simulink model "ThdRwRtStBkReclnTrgtPosSelc"  (R2018b)
settings: Solver=FixedStepDiscrete  StartTime=0.0  StopTime=10.0  RelTol=1e-3
undefined symbols (not defined in the file or in its folder): KeSMSw6sAcsEntryThdRwRtStBkReclnUpwdDnwdPos_Val, KeSMSw6sAcsEntryThdRwRtStBkReclnUpwdDnwdPosMax_Val, KeSMSw6sAcsEntryThdRwRtStBkReclnUpwdDnwdPosMin_Val, KeSMSw6sLugThdRwRtStBkReclnUpwdDnwdPos_Val, KeSMSw6sLugThdRwRtStBkReclnUpwdDnwdPosMax_Val, KeSMSw6sLugThdRwRtStBkReclnUpwdDnwdPosMin_Val, KeSMSw6sVIPThdRwRtStBkReclnUpwdDnwdPos_Val, KeSMSw6sVIPThdRwRtStBkReclnUpwdDnwdPosMax_Val, KeSMSw6sVIPThdRwRtStBkReclnUpwdDnwdPosMin_Val, KeSMSwAcsEntryThdRwRtStBkReclnUpwdDnwdPos_Val, KeSMSwAcsEntryThdRwRtStBkReclnUpwdDnwdPosMax_Val, KeSMSwAcsEntryThdRwRtStBkReclnUpwdDnwdPosMin_Val, KeSMSwAcsMd53ThdRwRtBkReclnUpwdDnwdPos_Val, KeSMSwAcsMd53ThdRwRtBkReclnUpwdDnwdPosMax_Val, KeSMSwAcsMd53ThdRwRtBkReclnUpwdDnwdPosMin_Val, KeSMSwLugThdRwRtStBkReclnUpwdDnwdPos_Val, KeSMSwLugThdRwRtStBkReclnUpwdDnwdPosMax_Val, KeSMSwLugThdRwRtStBkReclnUpwdDnwdPosMin_Val, KeSMSwVIPThdRwRtStBkReclnUpwdDnwdPos_Val, KeSMSwVIPThdRwRtStBkReclnUpwdDnwdPosMax_Val, KeSMSwVIPThdRwRtStBkReclnUpwdDnwdPosMin_Val
libraries: TrgtPosSelcLib x5
settings Model: Creator=sn2xws  LastModifiedBy=sn2xws
settings Model: ModifiedHistory=|
  | 2024.6.25
  | V3.0.0 557模式流程V1.6
settings DataIOCC: SaveFormat=StructureWithTime
settings OptimizationCC: DefaultParameterBehavior=Inlined  EnhancedBackFolding=on  PassReuseOutputArgsAs=Individual arguments  ZeroExternalMemoryAtStartup=off  ZeroInternalMemoryAtStartup=off  OptimizeBlockOrder=speed  DifferentSizesBufferReuse=on  OptimizationCustomize=off
settings DebuggingCC: ParameterTunabilityLossMsg=error
settings SFSimCC: MATLABDynamicMemAlloc=off
settings RTWCC: SystemTargetFile=autosar.tlc  GenCodeOnly=on  TemplateMakefile=ert_default_tmf  Description=AUTOSAR  GenerateReport=on  IncludeHyperlinkInReport=on  LaunchReport=on  GenerateTraceInfo=on  GenerateTraceReport=on  GenerateTraceReportSl=on  GenerateTraceReportSf=on  GenerateTraceReportEml=on  GenerateCodeMetricsReport=on
settings CodeAppCC: ForceParamTrailComments=on  IgnoreCustomStorageClasses=off  OperatorAnnotations=on  SimulinkDataObjDesc=on  SFDataObjDesc=on  InsertBlockDesc=on
settings STFCustomTargetCC: TargetLangStandard=C99 (ISO)  MultiwordLength=256  ParMdlRefBuildCompliant=on  CompOptLevelCompliant=on  IncludeMdlTerminateFcn=off  CombineOutputUpdateFcns=on  SuppressErrorStatus=on  ERTCustomFileBanners=on  SupportNonFinite=off  SupportComplex=off  SupportContinuousTime=off  SupportNonInlinedSFcns=off  RemoveResetFunc=on  MATLABClassNameForMDSCustomization=Simulink.SoftwareTarget.ERTCustomization  AutosarCompliant=on  UseToolchainInfoCompliant=on  LookupTableObjectStructAxisOrder=2,1,3,4,...  LUTObjectStructOrderEvenSpacing=Size,Table,Breakpoints  SystemTargetFile=autosar.tlc
settings ERTTargetCC: TargetLangStandard=C99 (ISO)  ConcurrentExecutionCompliant=off  IncludeMdlTerminateFcn=off  SuppressErrorStatus=on  SupportNonFinite=off  SupportComplex=off  ModelStepFunctionPrototypeControlCompliant=off  CPPClassGenCompliant=off  AutosarCompliant=on  LookupTableObjectStructAxisOrder=2,1,3,4,...  LUTObjectStructOrderEvenSpacing=Size,Table,Breakpoints  InlinedParameterPlacement=NonHierarchical  ERTCustomFileTemplate=example_file_process.tlc  ERTFilePackagingFormat=Compact

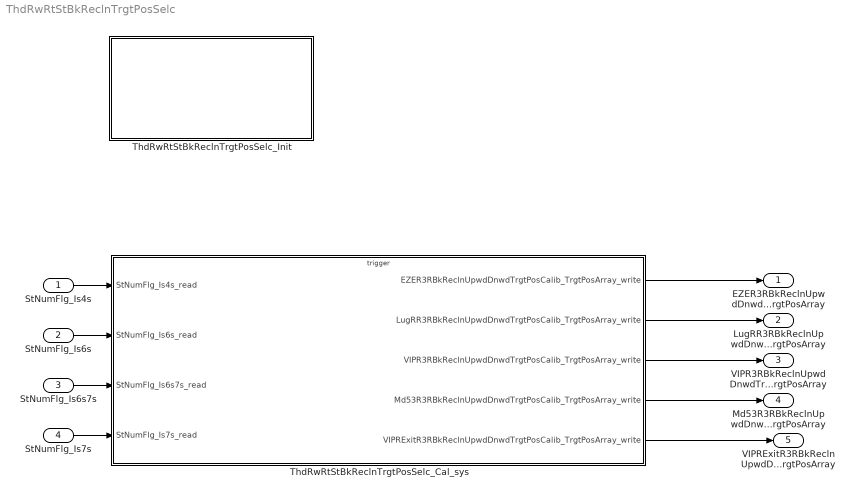
== system ThdRwRtStBkReclnTrgtPosSelc ==
  StNumFlg_Is4s : Inport  OutDataTypeStr=boolean  PortDimensions=1
  StNumFlg_Is6s : Inport  Port=2  OutDataTypeStr=boolean  PortDimensions=1
  StNumFlg_Is6s7s : Inport  Port=3  OutDataTypeStr=boolean  PortDimensions=1
  StNumFlg_Is7s : Inport  Port=4  OutDataTypeStr=boolean  PortDimensions=1
  ThdRwRtStBkReclnTrgtPosSelc_Cal_sys : Subsystem
  ThdRwRtStBkReclnTrgtPosSelc_Init : Subsystem
  EZER3RBkReclnUpwdDnwdTrgtPosCalib_TrgtPosArray : Outport  Description=|  OutDataTypeStr=uint16  PortDimensions=3
      | 0:Pos
      | 1:Max
      | 2:Min
  LugRR3RBkReclnUpwdDnwdTrgtPosCalib_TrgtPosArray : Outport  Description=|  Port=2  OutDataTypeStr=uint16  PortDimensions=3
      | 0:Pos
      | 1:Max
      | 2:Min
  VIPR3RBkReclnUpwdDnwdTrgtPosCalib_TrgtPosArray : Outport  Description=|  Port=3  OutDataTypeStr=uint16  PortDimensions=3
      | 0:Pos
      | 1:Max
      | 2:Min
  Md53R3RBkReclnUpwdDnwdTrgtPosCalib_TrgtPosArray : Outport  Description=|  Port=4  OutDataTypeStr=uint16  PortDimensions=3
      | 0:Pos
      | 1:Max
      | 2:Min
  VIPRExitR3RBkReclnUpwdDnwdTrgtPosCalib_TrgtPosArray : Outport  Description=|  Port=5  OutDataTypeStr=uint16  PortDimensions=3
      | 0:Pos
      | 1:Max
      | 2:Min
  wires:
  StNumFlg_Is4s/1 -> ThdRwRtStBkReclnTrgtPosSelc_Cal_sys/1(StNumFlg_Is4s_read)
  StNumFlg_Is6s/1 -> ThdRwRtStBkReclnTrgtPosSelc_Cal_sys/2(StNumFlg_Is6s_read)
  StNumFlg_Is6s7s/1 -> ThdRwRtStBkReclnTrgtPosSelc_Cal_sys/3(StNumFlg_Is6s7s_read)
  StNumFlg_Is7s/1 -> ThdRwRtStBkReclnTrgtPosSelc_Cal_sys/4(StNumFlg_Is7s_read)
  ThdRwRtStBkReclnTrgtPosSelc_Cal_sys/1(EZER3RBkReclnUpwdDnwdTrgtPosCalib_TrgtPosArray_write) -> EZER3RBkReclnUpwdDnwdTrgtPosCalib_TrgtPosArray/1
  ThdRwRtStBkReclnTrgtPosSelc_Cal_sys/2(LugRR3RBkReclnUpwdDnwdTrgtPosCalib_TrgtPosArray_write) -> LugRR3RBkReclnUpwdDnwdTrgtPosCalib_TrgtPosArray/1
  ThdRwRtStBkReclnTrgtPosSelc_Cal_sys/3(VIPR3RBkReclnUpwdDnwdTrgtPosCalib_TrgtPosArray_write) -> VIPR3RBkReclnUpwdDnwdTrgtPosCalib_TrgtPosArray/1
  ThdRwRtStBkReclnTrgtPosSelc_Cal_sys/4(Md53R3RBkReclnUpwdDnwdTrgtPosCalib_TrgtPosArray_write) -> Md53R3RBkReclnUpwdDnwdTrgtPosCalib_TrgtPosArray/1
  ThdRwRtStBkReclnTrgtPosSelc_Cal_sys/5(VIPRExitR3RBkReclnUpwdDnwdTrgtPosCalib_TrgtPosArray_write) -> VIPRExitR3RBkReclnUpwdDnwdTrgtPosCalib_TrgtPosArray/1

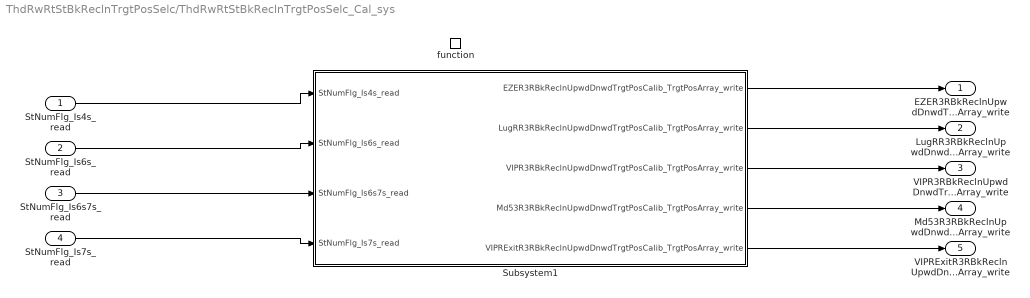
== system ThdRwRtStBkReclnTrgtPosSelc/ThdRwRtStBkReclnTrgtPosSelc_Cal_sys ==
  StNumFlg_Is4s_read : Inport
  StNumFlg_Is6s_read : Inport  Port=2
  StNumFlg_Is6s7s_read : Inport  Port=3
  StNumFlg_Is7s_read : Inport  Port=4
  function : TriggerPort  TriggerType=function-call  IsSimulinkFunction=on  FunctionName=ThdRwRtStBkReclnTrgtPosSelc_Cal  VariantControl=(inherit)
  Subsystem1 : Subsystem
  EZER3RBkReclnUpwdDnwdTrgtPosCalib_TrgtPosArray_write : Outport
      settings: EnsureOutportIsVirtual=on
  LugRR3RBkReclnUpwdDnwdTrgtPosCalib_TrgtPosArray_write : Outport  Port=2
      settings: EnsureOutportIsVirtual=on
  VIPR3RBkReclnUpwdDnwdTrgtPosCalib_TrgtPosArray_write : Outport  Port=3
      settings: EnsureOutportIsVirtual=on
  Md53R3RBkReclnUpwdDnwdTrgtPosCalib_TrgtPosArray_write : Outport  Port=4
      settings: EnsureOutportIsVirtual=on
  VIPRExitR3RBkReclnUpwdDnwdTrgtPosCalib_TrgtPosArray_write : Outport  Port=5
      settings: EnsureOutportIsVirtual=on
  wires:
  Subsystem1/1(EZER3RBkReclnUpwdDnwdTrgtPosCalib_TrgtPosArray_write) -> EZER3RBkReclnUpwdDnwdTrgtPosCalib_TrgtPosArray_write/1
  Subsystem1/2(LugRR3RBkReclnUpwdDnwdTrgtPosCalib_TrgtPosArray_write) -> LugRR3RBkReclnUpwdDnwdTrgtPosCalib_TrgtPosArray_write/1
  Subsystem1/3(VIPR3RBkReclnUpwdDnwdTrgtPosCalib_TrgtPosArray_write) -> VIPR3RBkReclnUpwdDnwdTrgtPosCalib_TrgtPosArray_write/1
  StNumFlg_Is7s_read/1 -> Subsystem1/4(StNumFlg_Is7s_read)
  StNumFlg_Is6s7s_read/1 -> Subsystem1/3(StNumFlg_Is6s7s_read)
  StNumFlg_Is6s_read/1 -> Subsystem1/2(StNumFlg_Is6s_read)
  StNumFlg_Is4s_read/1 -> Subsystem1/1(StNumFlg_Is4s_read)
  Subsystem1/4(Md53R3RBkReclnUpwdDnwdTrgtPosCalib_TrgtPosArray_write) -> Md53R3RBkReclnUpwdDnwdTrgtPosCalib_TrgtPosArray_write/1
  Subsystem1/5(VIPRExitR3RBkReclnUpwdDnwdTrgtPosCalib_TrgtPosArray_write) -> VIPRExitR3RBkReclnUpwdDnwdTrgtPosCalib_TrgtPosArray_write/1

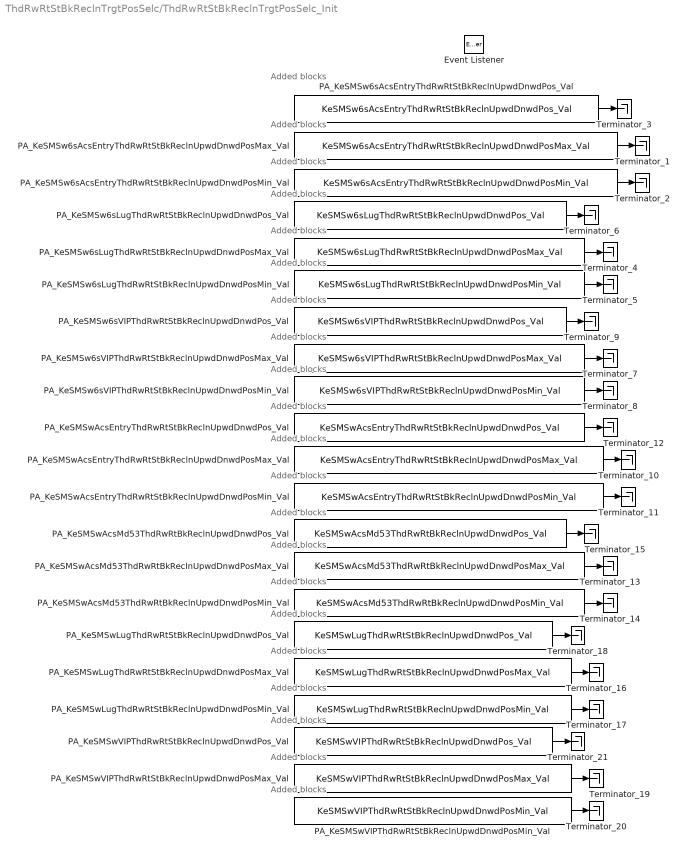
== system ThdRwRtStBkReclnTrgtPosSelc/ThdRwRtStBkReclnTrgtPosSelc_Init ==
  note: Added blocks
  note: Added blocks
  note: Added blocks
  note: Added blocks
  note: Added blocks
  note: Added blocks
  note: Added blocks
  note: Added blocks
  note: Added blocks
  note: Added blocks
  note: Added blocks
  note: Added blocks
  note: Added blocks
  note: Added blocks
  note: Added blocks
  note: Added blocks
  note: Added blocks
  note: Added blocks
  note: Added blocks
  note: Added blocks
  note: Added blocks
  Event Listener : EventListener  EventName=reset
  PA_KeSMSw6sAcsEntryThdRwRtStBkReclnUpwdDnwdPosMax_Val : Constant  Value=KeSMSw6sAcsEntryThdRwRtStBkReclnUpwdDnwdPosMax_Val
  PA_KeSMSw6sAcsEntryThdRwRtStBkReclnUpwdDnwdPosMin_Val : Constant  Value=KeSMSw6sAcsEntryThdRwRtStBkReclnUpwdDnwdPosMin_Val
  PA_KeSMSw6sAcsEntryThdRwRtStBkReclnUpwdDnwdPos_Val : Constant  Value=KeSMSw6sAcsEntryThdRwRtStBkReclnUpwdDnwdPos_Val
  PA_KeSMSw6sLugThdRwRtStBkReclnUpwdDnwdPosMax_Val : Constant  Value=KeSMSw6sLugThdRwRtStBkReclnUpwdDnwdPosMax_Val
  PA_KeSMSw6sLugThdRwRtStBkReclnUpwdDnwdPosMin_Val : Constant  Value=KeSMSw6sLugThdRwRtStBkReclnUpwdDnwdPosMin_Val
  PA_KeSMSw6sLugThdRwRtStBkReclnUpwdDnwdPos_Val : Constant  Value=KeSMSw6sLugThdRwRtStBkReclnUpwdDnwdPos_Val
  PA_KeSMSw6sVIPThdRwRtStBkReclnUpwdDnwdPosMax_Val : Constant  Value=KeSMSw6sVIPThdRwRtStBkReclnUpwdDnwdPosMax_Val
  PA_KeSMSw6sVIPThdRwRtStBkReclnUpwdDnwdPosMin_Val : Constant  Value=KeSMSw6sVIPThdRwRtStBkReclnUpwdDnwdPosMin_Val
  PA_KeSMSw6sVIPThdRwRtStBkReclnUpwdDnwdPos_Val : Constant  Value=KeSMSw6sVIPThdRwRtStBkReclnUpwdDnwdPos_Val
  PA_KeSMSwAcsEntryThdRwRtStBkReclnUpwdDnwdPosMax_Val : Constant  Value=KeSMSwAcsEntryThdRwRtStBkReclnUpwdDnwdPosMax_Val
  PA_KeSMSwAcsEntryThdRwRtStBkReclnUpwdDnwdPosMin_Val : Constant  Value=KeSMSwAcsEntryThdRwRtStBkReclnUpwdDnwdPosMin_Val
  PA_KeSMSwAcsEntryThdRwRtStBkReclnUpwdDnwdPos_Val : Constant  Value=KeSMSwAcsEntryThdRwRtStBkReclnUpwdDnwdPos_Val
  PA_KeSMSwAcsMd53ThdRwRtBkReclnUpwdDnwdPosMax_Val : Constant  Value=KeSMSwAcsMd53ThdRwRtBkReclnUpwdDnwdPosMax_Val
  PA_KeSMSwAcsMd53ThdRwRtBkReclnUpwdDnwdPosMin_Val : Constant  Value=KeSMSwAcsMd53ThdRwRtBkReclnUpwdDnwdPosMin_Val
  PA_KeSMSwAcsMd53ThdRwRtBkReclnUpwdDnwdPos_Val : Constant  Value=KeSMSwAcsMd53ThdRwRtBkReclnUpwdDnwdPos_Val
  PA_KeSMSwLugThdRwRtStBkReclnUpwdDnwdPosMax_Val : Constant  Value=KeSMSwLugThdRwRtStBkReclnUpwdDnwdPosMax_Val
  PA_KeSMSwLugThdRwRtStBkReclnUpwdDnwdPosMin_Val : Constant  Value=KeSMSwLugThdRwRtStBkReclnUpwdDnwdPosMin_Val
  PA_KeSMSwLugThdRwRtStBkReclnUpwdDnwdPos_Val : Constant  Value=KeSMSwLugThdRwRtStBkReclnUpwdDnwdPos_Val
  PA_KeSMSwVIPThdRwRtStBkReclnUpwdDnwdPosMax_Val : Constant  Value=KeSMSwVIPThdRwRtStBkReclnUpwdDnwdPosMax_Val
  PA_KeSMSwVIPThdRwRtStBkReclnUpwdDnwdPosMin_Val : Constant  Value=KeSMSwVIPThdRwRtStBkReclnUpwdDnwdPosMin_Val
  PA_KeSMSwVIPThdRwRtStBkReclnUpwdDnwdPos_Val : Constant  Value=KeSMSwVIPThdRwRtStBkReclnUpwdDnwdPos_Val
  Terminator_{1..21} (21 alike) : Terminator
  wires:
  PA_KeSMSw6sAcsEntryThdRwRtStBkReclnUpwdDnwdPosMax_Val/1 -> Terminator_1/1
  PA_KeSMSw6sAcsEntryThdRwRtStBkReclnUpwdDnwdPosMin_Val/1 -> Terminator_2/1
  PA_KeSMSw6sAcsEntryThdRwRtStBkReclnUpwdDnwdPos_Val/1 -> Terminator_3/1
  PA_KeSMSw6sLugThdRwRtStBkReclnUpwdDnwdPosMax_Val/1 -> Terminator_4/1
  PA_KeSMSw6sLugThdRwRtStBkReclnUpwdDnwdPosMin_Val/1 -> Terminator_5/1
  PA_KeSMSw6sLugThdRwRtStBkReclnUpwdDnwdPos_Val/1 -> Terminator_6/1
  PA_KeSMSw6sVIPThdRwRtStBkReclnUpwdDnwdPosMax_Val/1 -> Terminator_7/1
  PA_KeSMSw6sVIPThdRwRtStBkReclnUpwdDnwdPosMin_Val/1 -> Terminator_8/1
  PA_KeSMSw6sVIPThdRwRtStBkReclnUpwdDnwdPos_Val/1 -> Terminator_9/1
  PA_KeSMSwAcsEntryThdRwRtStBkReclnUpwdDnwdPosMax_Val/1 -> Terminator_10/1
  PA_KeSMSwAcsEntryThdRwRtStBkReclnUpwdDnwdPosMin_Val/1 -> Terminator_11/1
  PA_KeSMSwAcsEntryThdRwRtStBkReclnUpwdDnwdPos_Val/1 -> Terminator_12/1
  PA_KeSMSwAcsMd53ThdRwRtBkReclnUpwdDnwdPosMax_Val/1 -> Terminator_13/1
  PA_KeSMSwAcsMd53ThdRwRtBkReclnUpwdDnwdPosMin_Val/1 -> Terminator_14/1
  PA_KeSMSwAcsMd53ThdRwRtBkReclnUpwdDnwdPos_Val/1 -> Terminator_15/1
  PA_KeSMSwLugThdRwRtStBkReclnUpwdDnwdPosMax_Val/1 -> Terminator_16/1
  PA_KeSMSwLugThdRwRtStBkReclnUpwdDnwdPosMin_Val/1 -> Terminator_17/1
  PA_KeSMSwLugThdRwRtStBkReclnUpwdDnwdPos_Val/1 -> Terminator_18/1
  PA_KeSMSwVIPThdRwRtStBkReclnUpwdDnwdPosMax_Val/1 -> Terminator_19/1
  PA_KeSMSwVIPThdRwRtStBkReclnUpwdDnwdPosMin_Val/1 -> Terminator_20/1
  PA_KeSMSwVIPThdRwRtStBkReclnUpwdDnwdPos_Val/1 -> Terminator_21/1

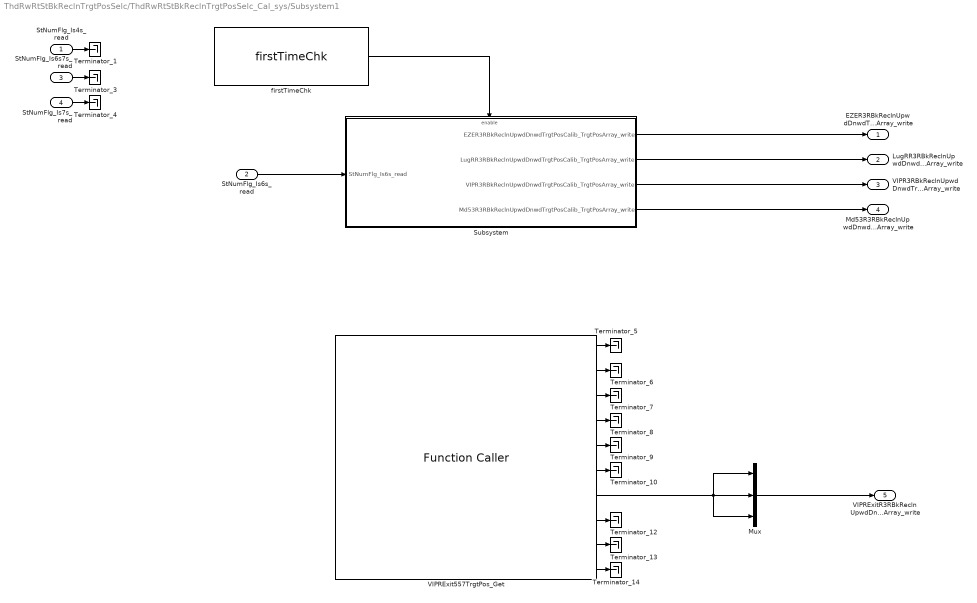
== system ThdRwRtStBkReclnTrgtPosSelc/ThdRwRtStBkReclnTrgtPosSelc_Cal_sys/Subsystem1 ==
  StNumFlg_Is4s_read : Inport
  StNumFlg_Is6s_read : Inport  Port=2
  StNumFlg_Is6s7s_read : Inport  Port=3
  StNumFlg_Is7s_read : Inport  Port=4
  Mux : Mux  Inputs=3
  Subsystem : Subsystem
  Terminator_{1,3..10,12..14} (12 alike) : Terminator
  VIPRExit557TrgtPos_Get : FunctionCaller  FunctionPrototype=[SecRwRtStBkReclnTrgtPos,SecRwRtStZeroTrgtPos,SecRwRtStLgrstUpwdDnwdTrgtPos,SecRwRtStLgrstInwdOtwdTrgtPos,ThdRwLtStBkReclnTrgtPos,ThdRwLtStFwdBkwdTrgtPos,ThdRwRtStBkReclnTrgtPos,ThdRwRtStFwdBkwdTrgtPos,PassStBkReclnTrgtPos,PassStFwdBkwdTrgtPos] = VIPRExit557TrgtPos_Get()  OutputArgumentSpecifications=uint16(1), uint16(1), uint16(1), uint16(1), uint16(1), uint16(1), uint16(1), uint16(1), uint16(1), uint16(1)
  firstTimeChk : TrgtPosSelcLib/firstTimeChk  SystemSampleTime=-1
  EZER3RBkReclnUpwdDnwdTrgtPosCalib_TrgtPosArray_write : Outport
      settings: EnsureOutportIsVirtual=on
  LugRR3RBkReclnUpwdDnwdTrgtPosCalib_TrgtPosArray_write : Outport  Port=2
      settings: EnsureOutportIsVirtual=on
  VIPR3RBkReclnUpwdDnwdTrgtPosCalib_TrgtPosArray_write : Outport  Port=3
      settings: EnsureOutportIsVirtual=on
  Md53R3RBkReclnUpwdDnwdTrgtPosCalib_TrgtPosArray_write : Outport  Port=4
      settings: EnsureOutportIsVirtual=on
  VIPRExitR3RBkReclnUpwdDnwdTrgtPosCalib_TrgtPosArray_write : Outport  Port=5
      settings: EnsureOutportIsVirtual=on
  wires:
  Subsystem/1(EZER3RBkReclnUpwdDnwdTrgtPosCalib_TrgtPosArray_write) -> EZER3RBkReclnUpwdDnwdTrgtPosCalib_TrgtPosArray_write/1
  StNumFlg_Is4s_read/1 -> Terminator_1/1
  firstTimeChk/1 -> Subsystem/Enable
  Subsystem/3(VIPR3RBkReclnUpwdDnwdTrgtPosCalib_TrgtPosArray_write) -> VIPR3RBkReclnUpwdDnwdTrgtPosCalib_TrgtPosArray_write/1
  StNumFlg_Is7s_read/1 -> Terminator_4/1
  Subsystem/2(LugRR3RBkReclnUpwdDnwdTrgtPosCalib_TrgtPosArray_write) -> LugRR3RBkReclnUpwdDnwdTrgtPosCalib_TrgtPosArray_write/1
  StNumFlg_Is6s_read/1 -> Subsystem/1(StNumFlg_Is6s_read)
  StNumFlg_Is6s7s_read/1 -> Terminator_3/1
  Subsystem/4(Md53R3RBkReclnUpwdDnwdTrgtPosCalib_TrgtPosArray_write) -> Md53R3RBkReclnUpwdDnwdTrgtPosCalib_TrgtPosArray_write/1
  VIPRExit557TrgtPos_Get/1 -> Terminator_5/1
  VIPRExit557TrgtPos_Get/2 -> Terminator_6/1
  VIPRExit557TrgtPos_Get/3 -> Terminator_7/1
  VIPRExit557TrgtPos_Get/4 -> Terminator_8/1
  VIPRExit557TrgtPos_Get/5 -> Terminator_9/1
  VIPRExit557TrgtPos_Get/6 -> Terminator_10/1
  VIPRExit557TrgtPos_Get/7 -> Mux/3, Mux/1, Mux/2
  VIPRExit557TrgtPos_Get/8 -> Terminator_12/1
  VIPRExit557TrgtPos_Get/9 -> Terminator_13/1
  VIPRExit557TrgtPos_Get/10 -> Terminator_14/1
  Mux/1 -> VIPRExitR3RBkReclnUpwdDnwdTrgtPosCalib_TrgtPosArray_write/1

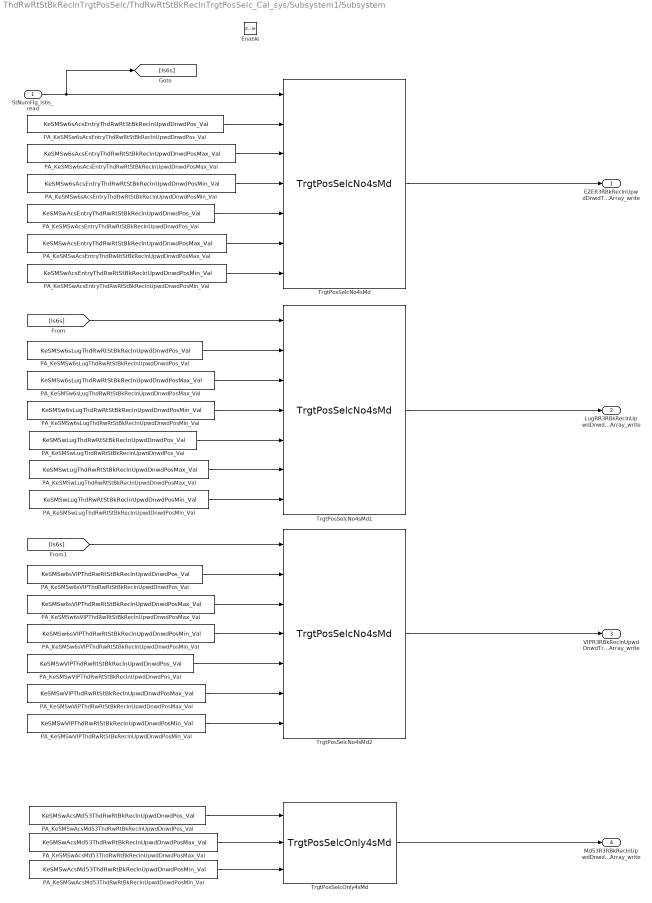
== system ThdRwRtStBkReclnTrgtPosSelc/ThdRwRtStBkReclnTrgtPosSelc_Cal_sys/Subsystem1/Subsystem ==
  StNumFlg_Is6s_read : Inport
  Enable : EnablePort
  PA_KeSMSw6sAcsEntryThdRwRtStBkReclnUpwdDnwdPosMax_Val : Constant  Value=KeSMSw6sAcsEntryThdRwRtStBkReclnUpwdDnwdPosMax_Val
  PA_KeSMSw6sAcsEntryThdRwRtStBkReclnUpwdDnwdPosMin_Val : Constant  Value=KeSMSw6sAcsEntryThdRwRtStBkReclnUpwdDnwdPosMin_Val
  PA_KeSMSw6sAcsEntryThdRwRtStBkReclnUpwdDnwdPos_Val : Constant  Value=KeSMSw6sAcsEntryThdRwRtStBkReclnUpwdDnwdPos_Val
  PA_KeSMSw6sLugThdRwRtStBkReclnUpwdDnwdPosMax_Val : Constant  Value=KeSMSw6sLugThdRwRtStBkReclnUpwdDnwdPosMax_Val
  PA_KeSMSw6sLugThdRwRtStBkReclnUpwdDnwdPosMin_Val : Constant  Value=KeSMSw6sLugThdRwRtStBkReclnUpwdDnwdPosMin_Val
  PA_KeSMSw6sLugThdRwRtStBkReclnUpwdDnwdPos_Val : Constant  Value=KeSMSw6sLugThdRwRtStBkReclnUpwdDnwdPos_Val
  PA_KeSMSw6sVIPThdRwRtStBkReclnUpwdDnwdPosMax_Val : Constant  Value=KeSMSw6sVIPThdRwRtStBkReclnUpwdDnwdPosMax_Val
  PA_KeSMSw6sVIPThdRwRtStBkReclnUpwdDnwdPosMin_Val : Constant  Value=KeSMSw6sVIPThdRwRtStBkReclnUpwdDnwdPosMin_Val
  PA_KeSMSw6sVIPThdRwRtStBkReclnUpwdDnwdPos_Val : Constant  Value=KeSMSw6sVIPThdRwRtStBkReclnUpwdDnwdPos_Val
  PA_KeSMSwAcsEntryThdRwRtStBkReclnUpwdDnwdPosMax_Val : Constant  Value=KeSMSwAcsEntryThdRwRtStBkReclnUpwdDnwdPosMax_Val
  PA_KeSMSwAcsEntryThdRwRtStBkReclnUpwdDnwdPosMin_Val : Constant  Value=KeSMSwAcsEntryThdRwRtStBkReclnUpwdDnwdPosMin_Val
  PA_KeSMSwAcsEntryThdRwRtStBkReclnUpwdDnwdPos_Val : Constant  Value=KeSMSwAcsEntryThdRwRtStBkReclnUpwdDnwdPos_Val
  PA_KeSMSwAcsMd53ThdRwRtBkReclnUpwdDnwdPosMax_Val : Constant  Value=KeSMSwAcsMd53ThdRwRtBkReclnUpwdDnwdPosMax_Val
  PA_KeSMSwAcsMd53ThdRwRtBkReclnUpwdDnwdPosMin_Val : Constant  Value=KeSMSwAcsMd53ThdRwRtBkReclnUpwdDnwdPosMin_Val
  PA_KeSMSwAcsMd53ThdRwRtBkReclnUpwdDnwdPos_Val : Constant  Value=KeSMSwAcsMd53ThdRwRtBkReclnUpwdDnwdPos_Val
  PA_KeSMSwLugThdRwRtStBkReclnUpwdDnwdPosMax_Val : Constant  Value=KeSMSwLugThdRwRtStBkReclnUpwdDnwdPosMax_Val
  PA_KeSMSwLugThdRwRtStBkReclnUpwdDnwdPosMin_Val : Constant  Value=KeSMSwLugThdRwRtStBkReclnUpwdDnwdPosMin_Val
  PA_KeSMSwLugThdRwRtStBkReclnUpwdDnwdPos_Val : Constant  Value=KeSMSwLugThdRwRtStBkReclnUpwdDnwdPos_Val
  PA_KeSMSwVIPThdRwRtStBkReclnUpwdDnwdPosMax_Val : Constant  Value=KeSMSwVIPThdRwRtStBkReclnUpwdDnwdPosMax_Val
  PA_KeSMSwVIPThdRwRtStBkReclnUpwdDnwdPosMin_Val : Constant  Value=KeSMSwVIPThdRwRtStBkReclnUpwdDnwdPosMin_Val
  PA_KeSMSwVIPThdRwRtStBkReclnUpwdDnwdPos_Val : Constant  Value=KeSMSwVIPThdRwRtStBkReclnUpwdDnwdPos_Val
  TrgtPosSelcNo4sMd : TrgtPosSelcLib/TrgtPosSelcNo4sMd  SystemSampleTime=-1
  TrgtPosSelcNo4sMd1 : TrgtPosSelcLib/TrgtPosSelcNo4sMd  SystemSampleTime=-1
  TrgtPosSelcNo4sMd2 : TrgtPosSelcLib/TrgtPosSelcNo4sMd  SystemSampleTime=-1
  TrgtPosSelcOnly4sMd : TrgtPosSelcLib/TrgtPosSelcOnly4sMd  SystemSampleTime=-1
  EZER3RBkReclnUpwdDnwdTrgtPosCalib_TrgtPosArray_write : Outport
      settings: EnsureOutportIsVirtual=on
  LugRR3RBkReclnUpwdDnwdTrgtPosCalib_TrgtPosArray_write : Outport  Port=2
      settings: EnsureOutportIsVirtual=on
  VIPR3RBkReclnUpwdDnwdTrgtPosCalib_TrgtPosArray_write : Outport  Port=3
      settings: EnsureOutportIsVirtual=on
  Md53R3RBkReclnUpwdDnwdTrgtPosCalib_TrgtPosArray_write : Outport  Port=4
      settings: EnsureOutportIsVirtual=on
  wires:
  TrgtPosSelcNo4sMd1/1 -> LugRR3RBkReclnUpwdDnwdTrgtPosCalib_TrgtPosArray_write/1
  StNumFlg_Is6s_read/1 -> [Is6s], TrgtPosSelcNo4sMd/1
  TrgtPosSelcNo4sMd/1 -> EZER3RBkReclnUpwdDnwdTrgtPosCalib_TrgtPosArray_write/1
  TrgtPosSelcNo4sMd2/1 -> VIPR3RBkReclnUpwdDnwdTrgtPosCalib_TrgtPosArray_write/1
  PA_KeSMSw6sAcsEntryThdRwRtStBkReclnUpwdDnwdPosMax_Val/1 -> TrgtPosSelcNo4sMd/3
  PA_KeSMSw6sAcsEntryThdRwRtStBkReclnUpwdDnwdPos_Val/1 -> TrgtPosSelcNo4sMd/2
  PA_KeSMSw6sAcsEntryThdRwRtStBkReclnUpwdDnwdPosMin_Val/1 -> TrgtPosSelcNo4sMd/4
  [Is6s] -> TrgtPosSelcNo4sMd1/1
  [Is6s] -> TrgtPosSelcNo4sMd2/1
  PA_KeSMSw6sLugThdRwRtStBkReclnUpwdDnwdPosMax_Val/1 -> TrgtPosSelcNo4sMd1/3
  PA_KeSMSw6sLugThdRwRtStBkReclnUpwdDnwdPos_Val/1 -> TrgtPosSelcNo4sMd1/2
  PA_KeSMSw6sLugThdRwRtStBkReclnUpwdDnwdPosMin_Val/1 -> TrgtPosSelcNo4sMd1/4
  PA_KeSMSw6sVIPThdRwRtStBkReclnUpwdDnwdPosMax_Val/1 -> TrgtPosSelcNo4sMd2/3
  PA_KeSMSw6sVIPThdRwRtStBkReclnUpwdDnwdPos_Val/1 -> TrgtPosSelcNo4sMd2/2
  PA_KeSMSw6sVIPThdRwRtStBkReclnUpwdDnwdPosMin_Val/1 -> TrgtPosSelcNo4sMd2/4
  PA_KeSMSwAcsEntryThdRwRtStBkReclnUpwdDnwdPosMax_Val/1 -> TrgtPosSelcNo4sMd/6
  PA_KeSMSwAcsEntryThdRwRtStBkReclnUpwdDnwdPos_Val/1 -> TrgtPosSelcNo4sMd/5
  PA_KeSMSwAcsEntryThdRwRtStBkReclnUpwdDnwdPosMin_Val/1 -> TrgtPosSelcNo4sMd/7
  PA_KeSMSwLugThdRwRtStBkReclnUpwdDnwdPosMax_Val/1 -> TrgtPosSelcNo4sMd1/6
  PA_KeSMSwLugThdRwRtStBkReclnUpwdDnwdPosMin_Val/1 -> TrgtPosSelcNo4sMd1/7
  PA_KeSMSwLugThdRwRtStBkReclnUpwdDnwdPos_Val/1 -> TrgtPosSelcNo4sMd1/5
  PA_KeSMSwVIPThdRwRtStBkReclnUpwdDnwdPosMax_Val/1 -> TrgtPosSelcNo4sMd2/6
  PA_KeSMSwVIPThdRwRtStBkReclnUpwdDnwdPos_Val/1 -> TrgtPosSelcNo4sMd2/5
  PA_KeSMSwVIPThdRwRtStBkReclnUpwdDnwdPosMin_Val/1 -> TrgtPosSelcNo4sMd2/7
  PA_KeSMSwAcsMd53ThdRwRtBkReclnUpwdDnwdPosMin_Val/1 -> TrgtPosSelcOnly4sMd/3
  PA_KeSMSwAcsMd53ThdRwRtBkReclnUpwdDnwdPosMax_Val/1 -> TrgtPosSelcOnly4sMd/2
  PA_KeSMSwAcsMd53ThdRwRtBkReclnUpwdDnwdPos_Val/1 -> TrgtPosSelcOnly4sMd/1
  TrgtPosSelcOnly4sMd/1 -> Md53R3RBkReclnUpwdDnwdTrgtPosCalib_TrgtPosArray_write/1
